simulink library "steppedLateralFlow_cl"  (R2022a)
settings: Solver=VariableStepAuto  StartTime=0.0  StopTime=10.0  RelTol=1e-3
undefined symbols (not defined in the file): env
settings Model: Creator=mcobb  LastModifiedBy=lhill8
settings SolverCC: AlgebraicLoopSolver=TrustRegion
settings DebuggingCC: UnconnectedInputMsg=warning  UnconnectedOutputMsg=warning  UnconnectedLineMsg=warning  SFMachineParentedDataDiag=warning  ArithmeticOperatorsInVariantConditions=warning
settings SFSimCC: CustomCodeUndefinedFunction=UseInterfaceOnly

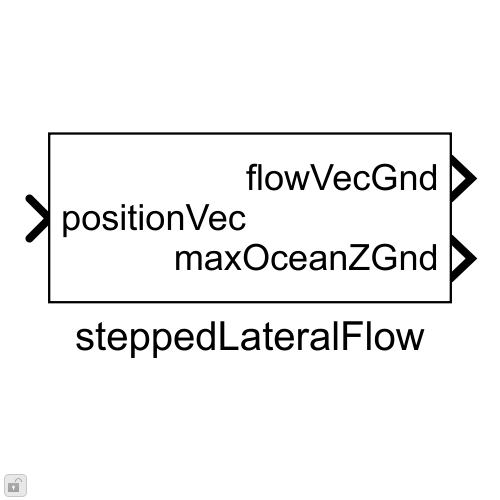
[thumbnail: Simulink's stored preview of the top-level diagram]
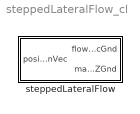
== system steppedLateralFlow_cl ==
  steppedLateralFlow : Subsystem

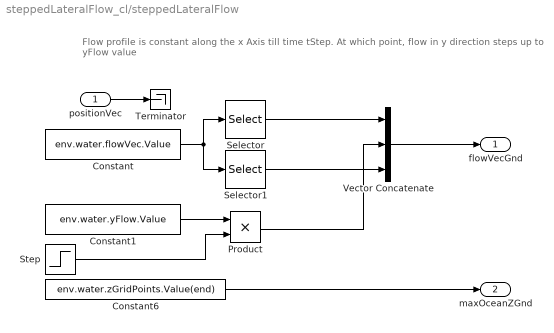
== system steppedLateralFlow_cl/steppedLateralFlow ==
  note: Flow profile is constant along the x Axis till time tStep. At which point, flow in y direction steps up to yFlow value
  positionVec : Inport
  Constant : Constant  Value=env.water.flowVec.Value
  Constant1 : Constant  Value=env.water.yFlow.Value
  Constant6 : Constant  Value=env.water.zGridPoints.Value(end)
  Product : Product
  Selector : Selector  InputPortWidth=3  IndexOptions=Index vector (dialog)  Indices=1  OutputSizes=1
  Selector1 : Selector  InputPortWidth=3  IndexOptions=Index vector (dialog)  Indices=3  OutputSizes=1
  Step : Step  Time=env.water.tStep.Value  SampleTime=0
  Terminator : Terminator
  Vector Concatenate : Concatenate  NumInputs=3
  flowVecGnd : Outport  VectorParamsAs1DForOutWhenUnconnected=off
  maxOceanZGnd : Outport  Port=2  VectorParamsAs1DForOutWhenUnconnected=off
  wires:
  positionVec/1 -> Terminator/1
  Constant/1 -> Selector1/1, Selector/1
  Selector/1 -> Vector Concatenate/1
  Constant6/1 -> maxOceanZGnd/1
  Vector Concatenate/1 -> flowVecGnd/1
  Constant1/1 -> Product/1
  Step/1 -> Product/2
  Product/1 -> Vector Concatenate/2
  Selector1/1 -> Vector Concatenate/3
